simulink model "varia_b"  (Simulink 5.0)
settings: Solver=ode45  StartTime=0.0  StopTime=40  RelTol=1e-3

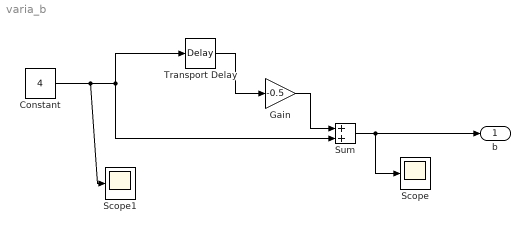
== system varia_b ==
  Constant : Constant  Value=4
  Gain : Gain  Gain=-0.5  SaturateOnIntegerOverflow=on
  Scope : Scope
  Scope1 : Scope
  Sum : Sum  SaturateOnIntegerOverflow=on
  Transport Delay : TransportDelay  DelayTime=20
  b : Outport
  wires:
  Constant/1 -> Sum/2, Transport Delay/1, Scope1/1
  Sum/1 -> Scope/1, b/1
  Transport Delay/1 -> Gain/1
  Gain/1 -> Sum/1
